simulink model "chap12_5sim"  (Simulink 8.3)
settings: Solver=ode45  StartTime=0.0  StopTime=20  FixedStep=0.001  RelTol=1e-3
settings Model: Creator=hp  LastModifiedBy=Prof_Liu  ExtModeTrigMode=oneshot  ExtModeArmWhenConnect=off
settings DataIOCC: LimitDataPoints=off  SignalLoggingName=sigsOut
settings OptimizationCC: BooleanDataType=off  ExpressionDepthLimit=2147483647  InitFltsAndDblsToZero=on
settings DebuggingCC: SaveWithParameterizedLinksMsg=none  SignalResolutionControl=TryResolveAllWithWarning  SolverPrmCheckMsg=none  MultiTaskDSMMsg=warning  MultiTaskCondExecSysMsg=none  FcnCallInpInsideContextMsg=UseLocalSettings
settings HardwareCC: TargetUnknown=on
settings RTWCC: IncludeERTFirstTime=on
settings GRTTargetCC: TargetFcnLib=ansi_tfl_tmw.mat

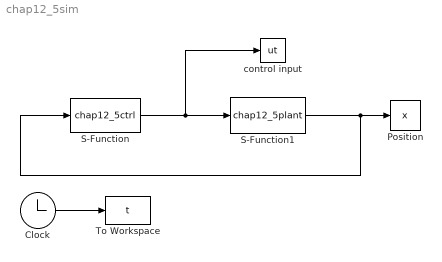
== system chap12_5sim ==
  Clock : Clock
  Position : ToWorkspace  VariableName=x  SampleTime=-1
  S-Function : S-Function  FunctionName=chap12_5ctrl  EnableBusSupport=off
  S-Function1 : S-Function  FunctionName=chap12_5plant  EnableBusSupport=off
  To Workspace : ToWorkspace  VariableName=t  SampleTime=-1
  control input : ToWorkspace  VariableName=ut  SampleTime=-1
  wires:
  S-Function/1 -> S-Function1/1, control input/1
  S-Function1/1 -> S-Function/1, Position/1
  Clock/1 -> To Workspace/1
